simulink model "BM_REF"  (R2023b)
settings: Solver=FixedStepDiscrete  StartTime=0.0  StopTime=10.0  FixedStep=0.01  RelTol=1e-3
undefined symbols (not defined in the file or in its folder): WAKEUP_SLEEP_REQ_E
libraries: simulink x4
settings Model: DataDictionary=BMS_MAIN.sldd  PauseTimes=0.9  Creator=Somashekar M  LastModifiedBy=Somashekar M

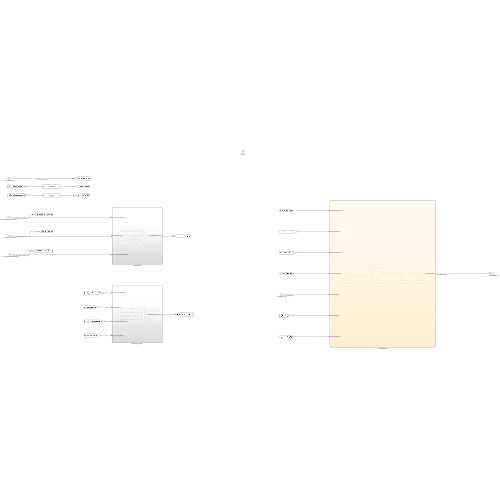
[thumbnail: Simulink's stored preview of the top-level diagram]
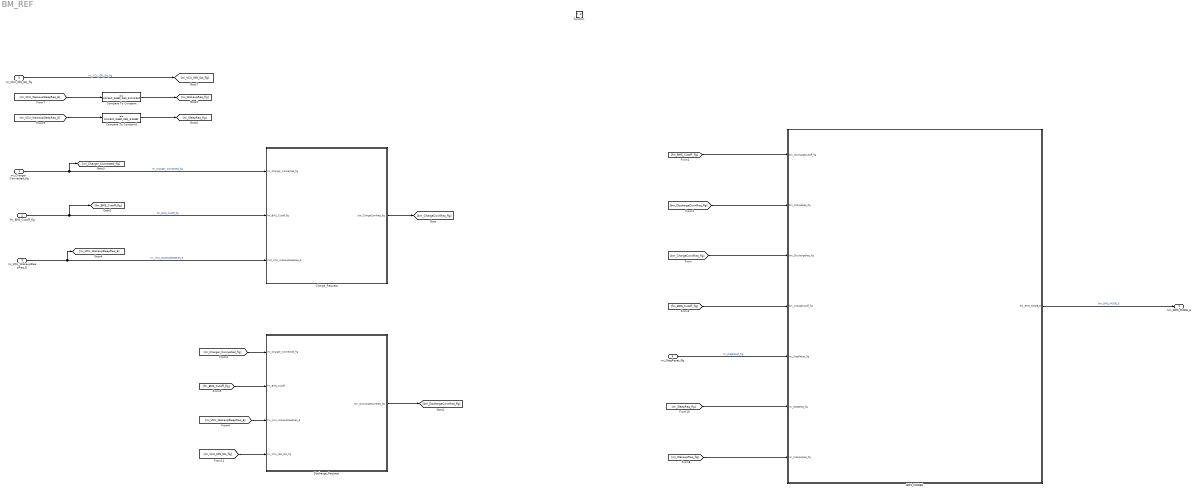
== system BM_REF ==
  mi_Charger_Connected_flg : Inport
  fm_BMS_Cutoff_flg : Inport  Port=2
  mi_VCU_WakeupSleepReq_E : Inport  Port=3
  mi_DiagReset_flg : Inport  Port=4
  mi_VCU_IGN_Sts_flg : Inport  Port=5
  function : TriggerPort  TriggerType=function-call  VariantControl=(inherit)
  BMS_MODES : Stateflow chart  TreatAsAtomicUnit=on
  Charge_Request : Subsystem
  Compare To Constant : simulink/Logic and Bit Operations/Compare To Constant  relop===  const=WAKEUP_SLEEP_REQ_E.WAKEUP  OutDataTypeStr=boolean
  Compare To Constant1 : simulink/Logic and Bit Operations/Compare To Constant  relop===  const=WAKEUP_SLEEP_REQ_E.SLEEP  OutDataTypeStr=boolean
  Discharge_Request : Subsystem
  bm_BMS_MODE_E : Outport
  wires:
  Discharge_Request/1(bm_DischargeConnReq_flg) -> [bm_DischargeConnReq_flg]
  Charge_Request/1(bm_ChargeConnReq_flg) -> [bm_ChargeConnReq_flg]
  [bm_DischargeConnReq_flg] -> BMS_MODES/2(bm_ChargeReq_flg)
  mi_Charger_Connected_flg/1 -> [mi_Charger_Connected_flg], Charge_Request/1(mi_Charger_Connected_flg)  "mi_Charger_Connected_flg"
  fm_BMS_Cutoff_flg/1 -> Charge_Request/2(fm_BMS_Cutoff_flg), [fm_BMS_Cutoff_flg]  "fm_BMS_Cutoff_flg"
  mi_VCU_WakeupSleepReq_E/1 -> [mi_VCU_WakeupSleepReq_E], Charge_Request/3(mid_VCU_WakeupSleepReq_E)  "mi_VCU_WakeupSleepReq_E"
  [bm_ChargeConnReq_flg] -> BMS_MODES/3(bm_DischargeReq_flg)
  [fm_BMS_Cutoff_flg] -> BMS_MODES/1(bm_DischargeCutoff_flg)
  [fm_BMS_Cutoff_flg] -> BMS_MODES/4(bm_ChargeCutoff_flg)
  mi_DiagReset_flg/1 -> BMS_MODES/5(mi_DiagReset_flg)  "mi_DiagReset_flg"
  [fm_BMS_Cutoff_flg] -> Discharge_Request/2(fm_BMS_Cutoff)
  [mi_Charger_Connected_flg] -> Discharge_Request/1(mi_Charger_Connected_flg)
  [mi_VCU_WakeupSleepReq_E] -> Discharge_Request/3(mi_VCU_WakeupSleepReq_E)
  [mi_SleepReq_flg] -> BMS_MODES/6(mi_SleepReq_flg)
  [mi_VCU_WakeupSleepReq_E] -> Compare To Constant/1
  Compare To Constant/1 -> [mi_WakeupReq_flg]
  Compare To Constant1/1 -> [mi_SleepReq_flg]
  [mi_VCU_WakeupSleepReq_E] -> Compare To Constant1/1
  BMS_MODES/1(bm_BMS_MODE_E) -> bm_BMS_MODE_E/1  "bm_BMS_MODE_E"
  mi_VCU_IGN_Sts_flg/1 -> [mi_VCU_IGN_Sts_flg]  "mi_VCU_IGN_Sts_flg"
  [mi_VCU_IGN_Sts_flg] -> Discharge_Request/4(mi_VCU_IGN_Sts_flg)
  [mi_WakeupReq_flg] -> BMS_MODES/7(mi_WakeupReq_flg)

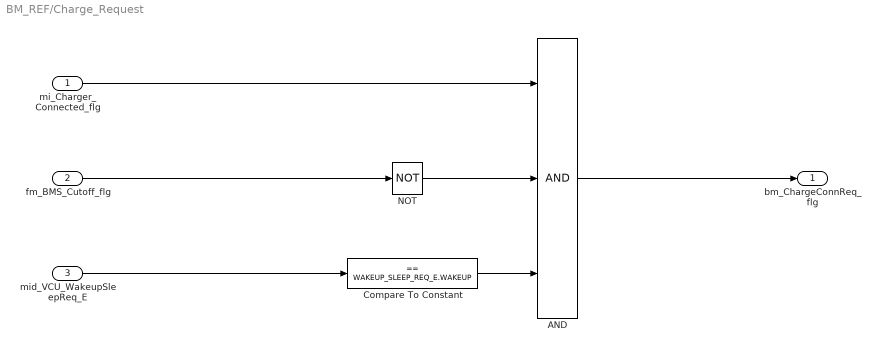
== system BM_REF/Charge_Request ==
  mi_Charger_Connected_flg : Inport
  fm_BMS_Cutoff_flg : Inport  Port=2
  mid_VCU_WakeupSleepReq_E : Inport  Port=3
  AND : Logic  Inputs=3  AllPortsSameDT=off  OutDataTypeStr=boolean
  Compare To Constant : simulink/Logic and Bit Operations/Compare To Constant  relop===  const=WAKEUP_SLEEP_REQ_E.WAKEUP  OutDataTypeStr=boolean
  NOT : Logic  Operator=NOT  IconShape=distinctive  AllPortsSameDT=off  OutDataTypeStr=boolean
  bm_ChargeConnReq_flg : Outport
  wires:
  AND/1 -> bm_ChargeConnReq_flg/1
  mi_Charger_Connected_flg/1 -> AND/1
  fm_BMS_Cutoff_flg/1 -> NOT/1
  NOT/1 -> AND/2
  mid_VCU_WakeupSleepReq_E/1 -> Compare To Constant/1
  Compare To Constant/1 -> AND/3

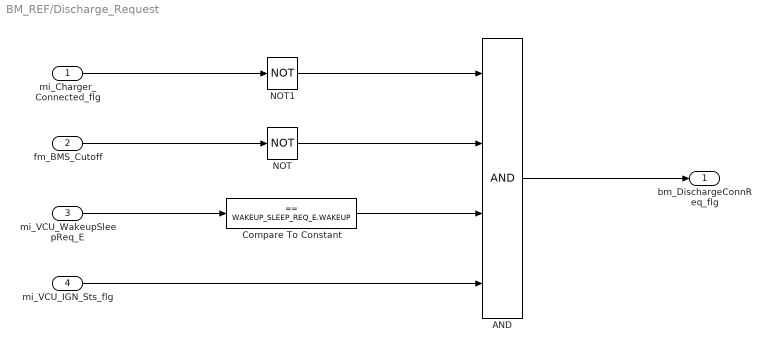
== system BM_REF/Discharge_Request ==
  mi_Charger_Connected_flg : Inport
  fm_BMS_Cutoff : Inport  Port=2
  mi_VCU_WakeupSleepReq_E : Inport  Port=3
  mi_VCU_IGN_Sts_flg : Inport  Port=4
  AND : Logic  Inputs=4  AllPortsSameDT=off  OutDataTypeStr=boolean
  Compare To Constant : simulink/Logic and Bit Operations/Compare To Constant  relop===  const=WAKEUP_SLEEP_REQ_E.WAKEUP  OutDataTypeStr=boolean
  NOT : Logic  Operator=NOT  IconShape=distinctive  AllPortsSameDT=off  OutDataTypeStr=boolean
  NOT1 : Logic  Operator=NOT  IconShape=distinctive  AllPortsSameDT=off  OutDataTypeStr=boolean
  bm_DischargeConnReq_flg : Outport
  wires:
  NOT/1 -> AND/2
  NOT1/1 -> AND/1
  mi_VCU_WakeupSleepReq_E/1 -> Compare To Constant/1
  fm_BMS_Cutoff/1 -> NOT/1
  mi_Charger_Connected_flg/1 -> NOT1/1
  Compare To Constant/1 -> AND/3
  mi_VCU_IGN_Sts_flg/1 -> AND/4
  AND/1 -> bm_DischargeConnReq_flg/1

== stateflow chart BM_REF/BMS_MODES ==
  state INITIALISE
    en:
    bm_BMS_MODE_E=BMS_MODES_E.INIT;
    standby_timer=0;
  state STANDBY
    en:
    bm_BMS_MODE_E=BMS_MODES_E.STANDBY;
    standby_timer=0;
    du:
    standby_timer=standby_timer+SAMPLE_TIME_10MS
  state Sleep_Pending
    en:
    bm_BMS_MODE_E=BMS_MODES_E.SLEEP_PENDING ;
    standby_timer=0;
  state CHARGE
    en:
    bm_BMS_MODE_E=BMS_MODES_E.CHARGE;
    standby_timer=0;
  state FAULT
    en:
    bm_BMS_MODE_E=BMS_MODES_E.FAULT;
    standby_timer=0;
  state DISCHARGE
    en:
    bm_BMS_MODE_E=BMS_MODES_E.DISCHARGE;
    standby_timer=0;
  state Sleep
    en:
    bm_BMS_MODE_E=BMS_MODES_E.SLEEP ;
    standby_timer=0;
  (default) -> INITIALISE
  INITIALISE -> STANDBY : [mi_WakeupReq_flg]
  Sleep_Pending -> STANDBY [order 1] : [mi_WakeupReq_flg ]
  STANDBY -> Sleep_Pending [order 2] : [mi_SleepReq_flg || standby_timer>=1000]
  STANDBY -> (junction 63) [order 1] : [bm_ChargeReq_flg]
  (junction 63) -> CHARGE
  STANDBY -> (junction 67) [order 3] : [bm_DischargeReq_flg]
  (junction 67) -> DISCHARGE
  (junction 75) -> STANDBY
  CHARGE -> (junction 75) [order 3] : [~bm_ChargeReq_flg]
  Sleep_Pending -> Sleep [order 2] : [after(1,sec)]
  Sleep -> Sleep_Pending : [mi_WakeupReq_flg]
  (junction 72) -> STANDBY
  DISCHARGE -> (junction 72) [order 2] : [~bm_DischargeReq_flg]
  FAULT -> STANDBY : [mi_DiagReset_flg]
  CHARGE -> FAULT [order 1] : [bm_ChargeCutoff_flg]
  DISCHARGE -> FAULT [order 1] : [bm_DischargeCutoff_flg]
  CHARGE -> (junction 101) [order 2] : [~bm_ChargeReq_flg && bm_DischargeReq_flg ]
  (junction 103) -> DISCHARGE
  (junction 101) -> (junction 103)
  data: bm_DischargeCutoff_flg input; bm_ChargeReq_flg input; bm_DischargeReq_flg input; bm_ChargeCutoff_flg input; mi_DiagReset_flg input; mi_SleepReq_flg input; mi_WakeupReq_flg input; bm_BMS_MODE_E output; standby_timer local uint16; SAMPLE_TIME_10MS parameter uint16
